simulink model "example_pipe_biflow"  (R2018b)
settings: Solver=VariableStepAuto  StartTime=0.0  StopTime=24*3600  RelTol=1e-3
undefined symbols (not defined in the file): path_carnot
libraries: carnot x5, simulink x2
settings Model: Creator=drhf  LastModifiedBy=P41573

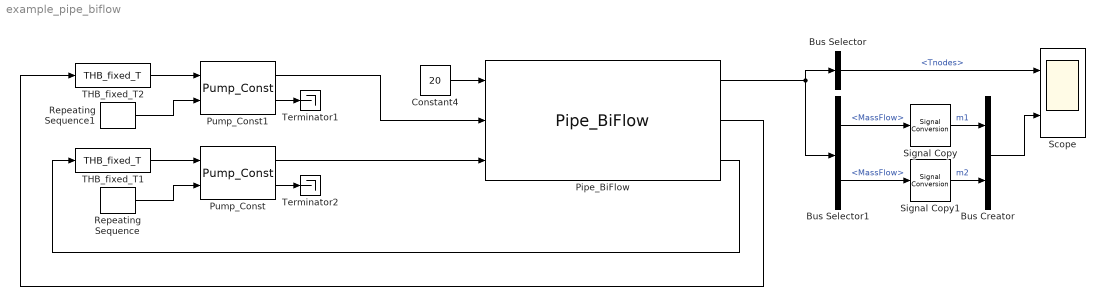
== system example_pipe_biflow ==
  Bus Creator : BusCreator  Inputs=2
  Bus Selector : BusSelector  OutputSignals=Tnodes
  Bus Selector1 : BusSelector  OutputSignals=THBout_pipe1.MassFlow,THBin_pipe2.MassFlow
  Constant4 : Constant  Value=20
  Pipe_BiFlow : carnot/Hydraulics/Pipe_BiFlow  t0=20  hgt=1273.2395  tini=[20 20 20 20 20 20 20 20 20 20]  mpts=[1 2 3 4 5 6 7 8 9 10]  PathName=fullfile(path_carnot('libsl'), 'Hydraulics', 'Pipe_Biflow', 'parameter_set')  FileName='PipeBF_set1.mat'  userPath=on  userParam=off  uwall=1  ubot=0  utop=0  axcond=1  volume=10  dia=0.1  standing=standing cylinder  nodes=10  mpoints=10  pipe1inlet=1  pipe1outlet=0  pipe1dia=0.1  pipe2inlet=0  pipe2outlet=1  pipe2dia=0.1
      settings: SourceProductName=Carnot
  Pump_Const : carnot/Hydraulics/Pump_Const  mdotmax=1800/3600  dia=0.02  p0=3e5  fluid_id=Water  mix=0  mix2=0  mix3=0  UA=3  mcp=4182  Tini=20  e0=10  e1=10  e2=-1
      settings: SourceProductName=Carnot
  Pump_Const1 : carnot/Hydraulics/Pump_Const  mdotmax=1200/3600  dia=0.02  p0=3e5  fluid_id=Water  mix=0  mix2=0  mix3=0  UA=3  mcp=4182  Tini=20  e0=10  e1=10  e2=-1
      settings: SourceProductName=Carnot
  Repeating Sequence : simulink/Sources/Repeating Sequence  rep_seq_t=[0 12.5 13.5 24]*3600  rep_seq_y=[1 1 0 0]
  Repeating Sequence1 : simulink/Sources/Repeating Sequence  rep_seq_t=[0 11.5 12.5 24]*3600  rep_seq_y=[0 0 1 1]
  Scope : Scope  NumInputPorts=2
  Signal Copy : SignalConversion  OverrideOpt=off
  Signal Copy1 : SignalConversion  OverrideOpt=off
  THB_fixed_T1 : carnot/Source/Simple/THB_fixed_T  t=60
      settings: SourceProductName=Carnot
  THB_fixed_T2 : carnot/Source/Simple/THB_fixed_T  t=40
      settings: SourceProductName=Carnot
  Terminator1 : Terminator
  Terminator2 : Terminator
  wires:
  THB_fixed_T1/1 -> Pump_Const/1
  Pump_Const/2 -> Terminator2/1
  Repeating Sequence/1 -> Pump_Const/2
  Constant4/1 -> Pipe_BiFlow/1
  Pipe_BiFlow/1 -> Bus Selector/1, Bus Selector1/1
  Repeating Sequence1/1 -> Pump_Const1/2
  Pump_Const1/2 -> Terminator1/1
  THB_fixed_T2/1 -> Pump_Const1/1
  Bus Selector/1 -> Scope/1  "<Tnodes>"
  Bus Selector1/1 -> Signal Copy/1  "<MassFlow>"
  Bus Selector1/2 -> Signal Copy1/1  "<MassFlow>"
  Signal Copy/1 -> Bus Creator/1  "m1"
  Signal Copy1/1 -> Bus Creator/2  "m2"
  Bus Creator/1 -> Scope/2
  Pump_Const/1 -> Pipe_BiFlow/3
  Pump_Const1/1 -> Pipe_BiFlow/2
  Pipe_BiFlow/2 -> THB_fixed_T2/1
  Pipe_BiFlow/3 -> THB_fixed_T1/1
